simulink library "threeWinches_cl"  (R2018b)
settings: Solver=VariableStepAuto  StartTime=0.0  StopTime=10.0  RelTol=1e-3
libraries: winch_ul x3
settings Model: Creator=mcobb  LastModifiedBy=mcobb

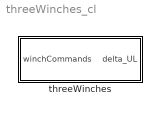
== system threeWinches_cl ==
  threeWinches : Subsystem  mask{maxSpeed=1, maxAccel=1, timeConst=1, tetherLengths=[100 100 100]}
      mask prompts: maxSpeed "Winch Max Speed"; maxAccel "Winch Max Acceleration"; timeConst "Winch Time Constant"; tetherLengths "Initial tether lengths"

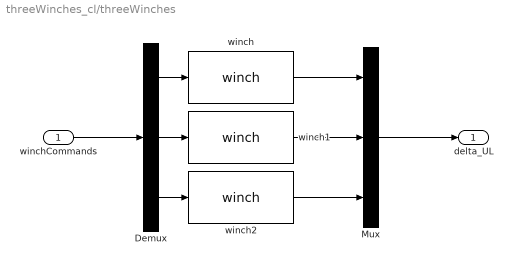
== system threeWinches_cl/threeWinches ==
  winchCommands : Inport
  Demux : Demux  Outputs=3
  Mux : Mux  Inputs=3
  winch : winch_ul/winch  initLength=tetherLengths(1)  maxSpd=maxSpeed(1)  tau=timeConst  maxAccl=maxAccel
  winch1 : winch_ul/winch  initLength=tetherLengths(2)  maxSpd=maxSpeed(2)  tau=timeConst  maxAccl=maxAccel
  winch2 : winch_ul/winch  initLength=tetherLengths(3)  maxSpd=maxSpeed(3)  tau=timeConst  maxAccl=maxAccel
  delta_UL : Outport
  wires:
  Demux/1 -> winch/1
  Mux/1 -> delta_UL/1
  Demux/2 -> winch1/1
  Demux/3 -> winch2/1
  winchCommands/1 -> Demux/1
  winch1/1 -> Mux/2
  winch/1 -> Mux/1
  winch2/1 -> Mux/3
